simulink model "keypad_template"  (R2020a)
settings: Solver=ode1  StartTime=0.0  StopTime=12  FixedStep=0.001  RelTol=1e-3  EnableMultiTasking=on
undefined symbols (not defined in the file or in its folder): sigbuilder_block
libraries: arduinolib x1
settings Model: ExtModeTrigDuration=2  Creator=estra  LastModifiedBy=Alexander Grebien
settings DataIOCC: ReturnWorkspaceOutputs=off
settings OptimizationCC: MaxStackSize=64  EfficientTunableParamExpr=on
settings DebuggingCC: ParameterTunabilityLossMsg=error  FrameProcessingCompatibilityMsg=warning  NonCurrentReleaseOperatingPointMsg=warning  ArithmeticOperatorsInVariantConditions=warning
settings HardwareCC: ProdBitPerInt=16  ProdBitPerPointer=16  ProdBitPerSizeT=16  ProdBitPerPtrDiffT=16  ProdLargestAtomicFloat=None  ProdWordSize=8  ProdHWDeviceType=Atmel->AVR
settings SFSimCC: SimUseLocalCustomCode=off  MATLABDynamicMemAlloc=off  CustomCodeUndefinedFunction=UseInterfaceOnly
settings RTWCC: SystemTargetFile=ert.tlc  HardwareBoard=Arduino Uno  TLCOptions=-aInlineSetEventsForThisBaseRateFcn=TLC_FALSE -aSuppressMultiTaskScheduler=TLC_FALSE -aRateBasedStepFcn=1  TemplateMakefile=ert_default_tmf  GenerateReport=on  RTWUseLocalCustomCode=off  Toolchain=Arduino AVR  BuildConfiguration=Faster Runs  IncludeHyperlinkInReport=on  LaunchReport=on  GenerateTraceInfo=on  GenerateTraceReport=on  GenerateTraceReportSl=on  GenerateTraceReportSf=on  GenerateTraceReportEml=on
settings CodeAppCC: ForceParamTrailComments=on  IgnoreCustomStorageClasses=off  OperatorAnnotations=on  SimulinkDataObjDesc=on  SFDataObjDesc=on  MATLABFcnDesc=on  InsertBlockDesc=on  StateflowObjectComments=on  MATLABSourceComments=on
settings ERTTargetCC: MultiwordLength=2048  SupportContinuousTime=on  SupportVariableSizeSignals=on

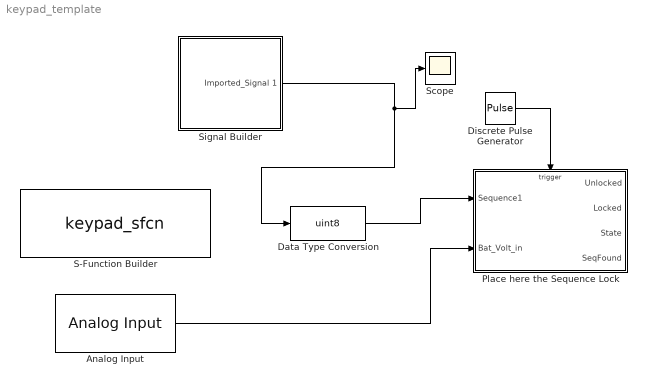
== system keypad_template ==
  Analog Input : arduinolib/Analog Input  pinNumber=4  ReadResultsOnly=off  ConversionTriggerSource=Software  ExternalTriggerType=uint32( 0 )  OutputDataType=uint16  EnableConversionCompleteNotify=off  EnableOuputStatus=off  SampleTime=1  blockPlatform=arduino
  Data Type Conversion : DataTypeConversion  OutDataTypeStr=uint8
  Discrete Pulse Generator : DiscretePulseGenerator  PulseType=Time based  Period=0.01  PulseWidth=50
  Place here the Sequence Lock : Subsystem
  S-Function Builder : S-Function  InitFcn=try, set_param(gcb,'FunctionName','keypad_sfcn'), end  FunctionName=keypad_sfcn  SFunctionModules=keypad_sfcn_wrapper  SFunctionDeploymentMode=off  EnableBusSupport=off  mask(S-Function Builder){}
      mask help: Simulink:masks:SFunctionBuilder_MD
      mask init:
      | val = [[.9  0.75 0.75 1 1 .9 .9 1]',[1 1 0.75 0.75 .9 .9 1 .9]'];try , sys = get_param(gcb,'SfunBuilderFcnName');if isempty(sys), sys = get_param(gcb,'FunctionName'); end,catch, sys = get_param(gcb,'FunctionName'); end
      settings: CopyFcn=set_param(gcbh,'LinkStatus','none')  PreSaveFcn=try, set_param(gcb,'FunctionName','keypad_sfcn'), end  OpenFcn=sfunctionwizard(gcbh)
      mask Display: plot(val(:,1),val(:,2)),disp(sys), port_label('output',1,'y0')
  Scope : Scope
  Signal Builder : Subsystem  Tag=STV Subsys  LoadFcn=sigbuilder_block('load');  StartFcn=sigbuilder_block('start');  StopFcn=sigbuilder_block('stop');  ClipboardFcn=sigbuilder_block('clipboard');  mask(Sigbuilder block){tuvar=[0:10]}
      mask help: Simulink:masks:SigbuilderBlock_MD
      mask init:
      | if ~strcmp(get_param(bdroot(gcbh),'SimulationStatus'),'stopped') tuvar = sigbuilder_block('maskInit'); end
      settings: CopyFcn=sigbuilder_block('copy');  DeleteFcn=sigbuilder_block('delete');  ModelCloseFcn=sigbuilder_block('modelClose');  PreSaveFcn=sigbuilder_block('preSave');  PauseFcn=sigbuilder_block('pause');  ContinueFcn=sigbuilder_block('continue');  NameChangeFcn=sigbuilder_block('namechange');  OpenFcn=sigbuilder_block('open',[437.6 199.2 550.4 400 ]);  CloseFcn=sigbuilder_block('close');
      mask Display: plot(0, 0, 100, 100,[2, 2, 32, 32, 2], [68, 8, 8, 68, 68],[32, 2], [38, 38], [32, 19, 2],[53, 60, 44], [32, 17, 17, 2],[16, 16, 31, 31]);txt = getActiveGroup(gcbh);text(2, 100, txt,'verticalAlignment', 'top');
  wires:
  Signal Builder/1(Imported_Signal 1) -> Data Type Conversion/1, Scope/1
  Data Type Conversion/1 -> Place here the Sequence Lock/1(Sequence1)
  Discrete Pulse Generator/1 -> Place here the Sequence Lock/Trigger
  Analog Input/1 -> Place here the Sequence Lock/2(Bat_Volt_in)

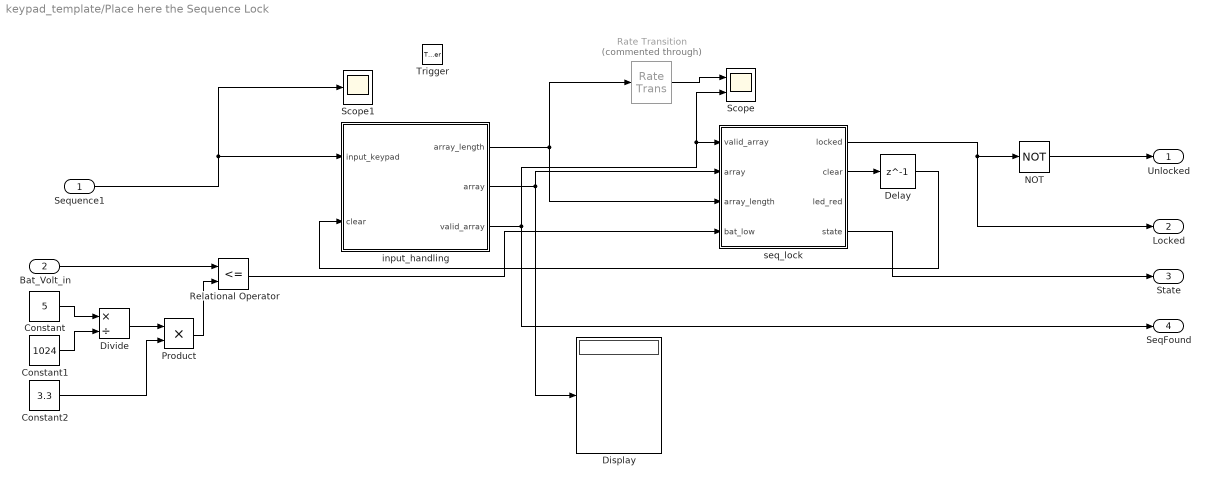
== system keypad_template/Place here the Sequence Lock ==
  Sequence1 : Inport
  Bat_Volt_in : Inport  Port=2
  Trigger : TriggerPort  VariantControl=Variant  PortDimensions=1
  Constant : Constant  Value=5
  Constant1 : Constant  Value=1024
  Constant2 : Constant  Value=3.3
  Delay : Delay  DelayLength=1  InitialCondition=0
  Display : Display
  Divide : Product  Inputs=*/
  NOT : Logic  Operator=NOT  IconShape=distinctive  AllPortsSameDT=off  OutDataTypeStr=boolean
  Product : Product
  Rate Transition : RateTransition  Commented=through  OutPortSampleTimeOpt=Multiple of input port sample time  OutPortSampleTimeMultiple=50  OutPortSampleTime=1
  Relational Operator : RelationalOperator  Operator=<=  OutDataTypeStr=boolean  RndMeth=Simplest
  Scope : Scope  NumInputPorts=2
  Scope1 : Scope
  input_handling : Stateflow chart  TreatAsAtomicUnit=on
  seq_lock : Stateflow chart  TreatAsAtomicUnit=on
  Unlocked : Outport  VectorParamsAs1DForOutWhenUnconnected=off
  Locked : Outport  Port=2  VectorParamsAs1DForOutWhenUnconnected=off
  State : Outport  Port=3  VectorParamsAs1DForOutWhenUnconnected=off
  SeqFound : Outport  Port=4  VectorParamsAs1DForOutWhenUnconnected=off
  wires:
  input_handling/2(array) -> seq_lock/2(array), Display/1
  Rate Transition/1 -> Scope/1
  seq_lock/1(locked) -> NOT/1, Locked/1
  input_handling/1(array_length) -> seq_lock/3(array_length), Rate Transition/1
  input_handling/3(valid_array) -> SeqFound/1, Scope/2, seq_lock/1(valid_array)
  NOT/1 -> Unlocked/1
  seq_lock/4(state) -> State/1
  seq_lock/2(clear) -> Delay/1
  Delay/1 -> input_handling/2(clear)
  Sequence1/1 -> Scope1/1, input_handling/1(input_keypad)
  Bat_Volt_in/1 -> Relational Operator/1
  Constant1/1 -> Divide/2
  Constant/1 -> Divide/1
  Divide/1 -> Product/1
  Constant2/1 -> Product/2
  Product/1 -> Relational Operator/2
  Relational Operator/1 -> seq_lock/4(bat_low)

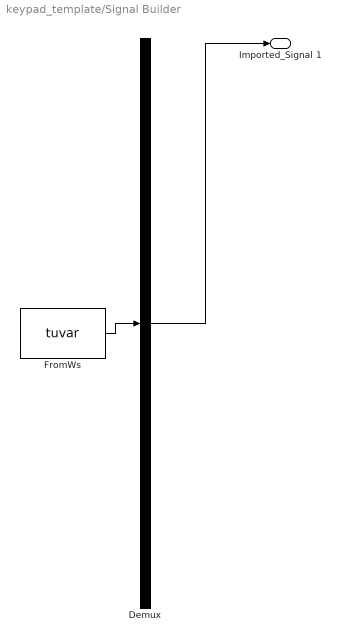
== system keypad_template/Signal Builder ==
  Demux : Demux  Tag=STV Demux  Outputs=1
      settings: DisplayOption=none
  FromWs : FromWorkspace  Tag=STV FromWs  VariableName=tuvar
      SigBuilderData=|
      | common.afterFinalStr = 'Extrapolate'
      | common.sampleTime = 0
      | dataSet.timeRange = [0 7]
      | dataSet.name = 'Imported_Group 1'
      | sbobj.Groups.Name = 'Imported_Group 1'
      | sbobj.Groups.Signals.Name = 'Imported_Signal 1'
      | sbobj.Groups.Signals.XData = [0 1 1 1.01 1.01 2 2 2.01 2.01 3 3 3.01 3.01 4 4 4.01 4.01 5 5 5.01 5.01 6 6 6.01 6.01 7]
      | sbobj.Groups.Signals.YData = [0 0 49 49 0 0 48 48 0 0 48 48 0 0 49 49 0 0 50 50 0 0 42 42 0 0]
      | sbobj.Groups.TimeRange = [0 6.01]
  Imported_Signal 1 : Outport  Tag=STV Outport
  wires:
  Demux/1 -> Imported_Signal 1/1
  FromWs/1 -> Demux/1

== stateflow chart keypad_template/Place here the Sequence Lock/input_handling ==
  settings: updateMethod=DISCRETE
  state INIT
    array_length = 0;
    array = uint8([]);
    valid_array = false;
  state CONCATENATE
    entry:
    array_length = uint8(length(array));
    array = cat(1, array, input_keypad);
    during:
    exit:
  state IDLE
    %Do absolutely nothing :D
  state STRING_FINSHED
    entry:
    valid_array = true;
    array_length = uint8(length(array));
    during:
    exit:
  (default) -> INIT
  IDLE -> INIT [order 2] : [after(7,sec) || clear==true]
  CONCATENATE -> INIT [order 1] : [array_length > 7]
  INIT -> IDLE [order 1] : [input_keypad == 0]
  INIT -> CONCATENATE [order 2]
  IDLE -> CONCATENATE [order 1] : [(input_keypad <= '9' && input_keypad >= '0') || input_keypad == '*'|| input_keypad == '#']
  CONCATENATE -> (junction 32) [order 3] : [hasChangedTo(input_keypad,uint8(0))]
  CONCATENATE -> STRING_FINSHED [order 2] : [(input_keypad=='*' || input_keypad=='#') && array_length >= 2]
  (junction 32) -> IDLE
  STRING_FINSHED -> (junction 32) : [hasChangedTo(input_keypad,uint8(0))]
  data: input_keypad input uint8 size=1 [0..254]; array_length output uint8 size=1; array output uint8 size=9; clear input boolean size=1; valid_array output boolean size=1

== stateflow chart keypad_template/Place here the Sequence Lock/seq_lock ==
  state INIT
    locked = false;
    clear = false;
    keep_password = false;
    state=0;
  state IDLE
    clear = false;
    locked = false;
  state LOCKED
    if(keep_password)
    password = password_old;
    else
    password = array;
    end
    password_length = uint8(length(password));
    clear = false;
    led_red = clear;
    locked = true;
  state WRONG_PASS
    %led_red blinken
    clear = true;
    led_red = clear;
  state UNLOCKED
    password_old = password;
    locked = false;
    keep_password = false;
  (default) -> INIT
  INIT -> IDLE
  (junction 65) -> IDLE [order 2] : {keep_password = false}
  IDLE -> LOCKED : [valid_array && (array(1) == '*') && (~(array(2) == '*'))]
  (junction 65) -> LOCKED [order 1] : [(array(1) == '*') && (array(2) == '*')]{keep_password = true}
  UNLOCKED -> (junction 65) : [valid_array]
  WRONG_PASS -> LOCKED : [after(3,sec)]
  LOCKED -> (junction 26) : [array_length == password_length]
  (junction 26) -> WRONG_PASS [order 2] : [compare(array, array_length, password, password_length) == 0]
  (junction 26) -> UNLOCKED [order 1] : [compare(array, array_length, password, password_length) == 1]
  data: password local uint8 size=9; locked output boolean size=1; valid_array input boolean size=1; array input uint8 size=9; array_length input uint8 size=1; clear output boolean size=1; password_length local uint8 size=1; password_old local uint8 size=9; led_red output boolean size=1; keep_password local boolean size=1; state output uint8 size=1; bat_low input boolean
